simulink library "merge_control_lib"  (Simulink 8.2)
settings: Solver=ode1  StartTime=0.0  StopTime=Inf  FixedStep=0.001  RelTol=1e-3
PostLoadFcn:
  | , if any(exist('dsrtsu_mdlpostloadfcn', 'file') == [2, 3, 6]), try dsrtsu_mdlpostloadfcn('Execute', bdroot); catch fprintf('Error in PostLoadFcn (dsrtsu_mdlpostloadfcn) for model "%s":\n %s\n', bdroot, lasterr); end, end,
libraries: merge_control_lib x6, simulink x4
settings Model: DSRTSU_INTERNAL_RTI_VER=450  DSRTSU_INTERNAL_RTI_TYPE=rti1401  DSRTSU_INTERNAL_RTIFPGA=40  Creator=rushk1  LastModifiedBy=rushk1

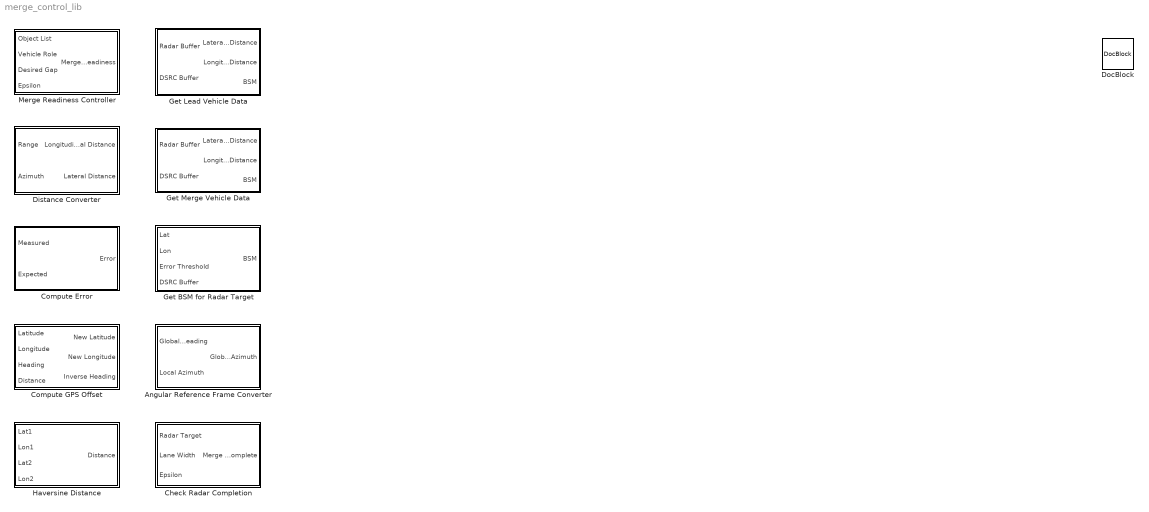
== system merge_control_lib ==
  Angular Reference Frame Converter : Subsystem
  Check Radar Completion : Subsystem
  Compute Error : Subsystem
  Compute GPS Offset : Subsystem
  Distance Converter : Subsystem  TreatAsAtomicUnit=on
      settings: RTWFcnNameOpts=Use subsystem name  RTWFileNameOpts=Use function name
  DocBlock : simulink/Model-Wide Utilities/DocBlock  DocumentType=Text
  Get BSM for Radar Target : Subsystem
  Get Lead Vehicle Data : Subsystem
  Get Merge Vehicle Data : Subsystem
  Haversine Distance : Subsystem
  Merge Readiness Controller : Subsystem

== system merge_control_lib/Angular Reference Frame Converter ==
  Global Heading : Inport
  Local Azimuth : Inport  Port=2
  Degrees in Circle : Constant  Value=360
  Math Function : Math  Operator=mod  OutputSignalType=real  SaturateOnIntegerOverflow=on
  Sum : Sum  Inputs=|++
  Global Azimuth : Outport
  wires:
  Local Azimuth/1 -> Sum/2
  Global Heading/1 -> Sum/1
  Sum/1 -> Math Function/1
  Math Function/1 -> Global Azimuth/1
  Degrees in Circle/1 -> Math Function/2

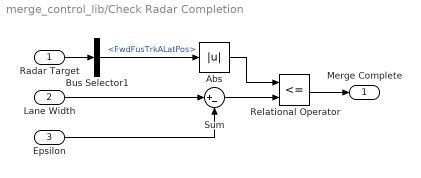
== system merge_control_lib/Check Radar Completion ==
  Radar Target : Inport  OutDataTypeStr=Bus: FusObjectTrackA
  Lane Width : Inport  Port=2  OutDataTypeStr=double
  Epsilon : Inport  Port=3  OutDataTypeStr=double
  Abs : Abs
  Bus Selector1 : BusSelector  OutputSignals=FwdFusTrkALatPos
  Relational Operator : RelationalOperator  Operator=<=  OutDataTypeStr=boolean
  Sum : Sum  Inputs=|+-
  Merge Complete : Outport
  wires:
  Radar Target/1 -> Bus Selector1/1
  Bus Selector1/1 -> Abs/1  "<FwdFusTrkALatPos>"
  Lane Width/1 -> Sum/1
  Relational Operator/1 -> Merge Complete/1
  Abs/1 -> Relational Operator/1
  Sum/1 -> Relational Operator/2
  Epsilon/1 -> Sum/2

== system merge_control_lib/Compute Error ==
  Measured : Inport
  Expected : Inport  Port=2
  Abs : Abs
  Subtract : Sum  Inputs=+-
  Error : Outport
  wires:
  Measured/1 -> Subtract/1
  Expected/1 -> Subtract/2
  Subtract/1 -> Abs/1
  Abs/1 -> Error/1

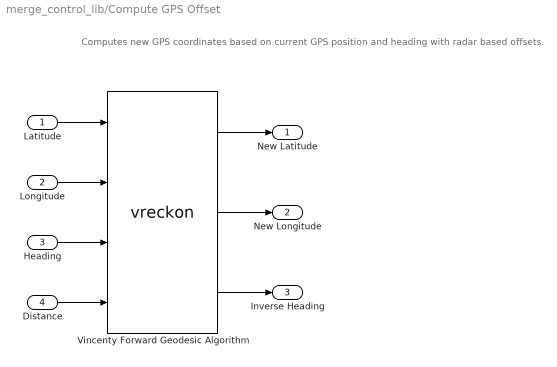
== system merge_control_lib/Compute GPS Offset ==
  note: Computes new GPS coordinates based on current GPS position and heading with radar based offsets.
  Latitude : Inport
  Longitude : Inport  Port=2
  Heading : Inport  Port=3
  Distance : Inport  Port=4
  Vincenty Forward Geodesic Algorithm : M-S-Function  FunctionName=vreckon
  New Latitude : Outport
  New Longitude : Outport  Port=2
  Inverse Heading : Outport  Port=3
  wires:
  Latitude/1 -> Vincenty Forward Geodesic Algorithm/1
  Longitude/1 -> Vincenty Forward Geodesic Algorithm/2
  Distance/1 -> Vincenty Forward Geodesic Algorithm/4
  Heading/1 -> Vincenty Forward Geodesic Algorithm/3
  Vincenty Forward Geodesic Algorithm/1 -> New Latitude/1
  Vincenty Forward Geodesic Algorithm/2 -> New Longitude/1
  Vincenty Forward Geodesic Algorithm/3 -> Inverse Heading/1

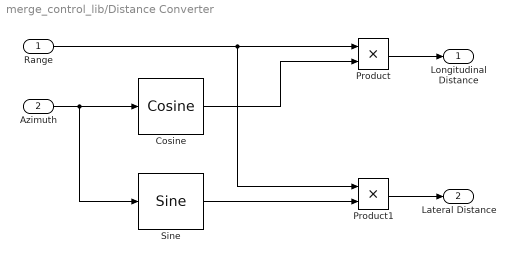
== system merge_control_lib/Distance Converter ==
  Range : Inport
  Azimuth : Inport  Port=2
  Cosine : simulink/Lookup Tables/Cosine  Formula=cos(2*pi*u)  NumDataPoints=(2^5)+1  OutputWordLength=16  InternalRulePriority=Speed
  Product : Product
  Product1 : Product
  Sine : simulink/Lookup Tables/Sine  Formula=sin(2*pi*u)  NumDataPoints=(2^5)+1  OutputWordLength=16  InternalRulePriority=Speed
  Longitudinal Distance : Outport
  Lateral Distance : Outport  Port=2
  wires:
  Product/1 -> Longitudinal Distance/1
  Azimuth/1 -> Sine/1, Cosine/1
  Cosine/1 -> Product/2
  Range/1 -> Product1/1, Product/1
  Product1/1 -> Lateral Distance/1
  Sine/1 -> Product1/2

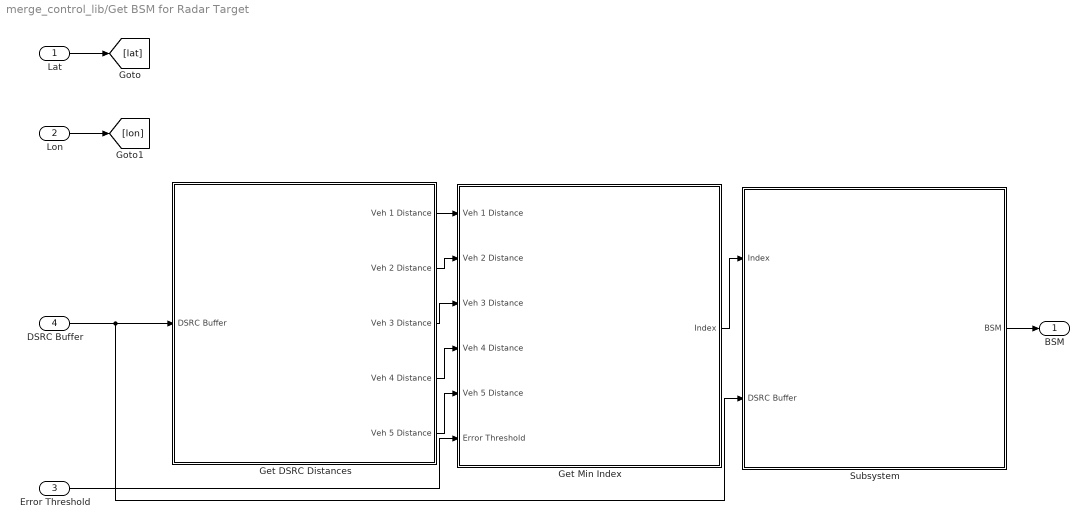
== system merge_control_lib/Get BSM for Radar Target ==
  Lat : Inport
  Lon : Inport  Port=2
  Error Threshold : Inport  Port=3
  DSRC Buffer : Inport  Port=4  OutDataTypeStr=Bus: BSMStoreBus
  Get DSRC Distances : Subsystem
  Get Min Index : Subsystem
  Subsystem : Subsystem
  BSM : Outport
  wires:
  Lat/1 -> [lat]
  Lon/1 -> [lon]
  DSRC Buffer/1 -> Subsystem/2(DSRC Buffer), Get DSRC Distances/1(DSRC Buffer)
  Get DSRC Distances/1(Veh 1 Distance) -> Get Min Index/1(Veh 1 Distance)
  Get DSRC Distances/4(Veh 4 Distance) -> Get Min Index/4(Veh 4 Distance)
  Get DSRC Distances/2(Veh 2 Distance) -> Get Min Index/2(Veh 2 Distance)
  Get DSRC Distances/5(Veh 5 Distance) -> Get Min Index/5(Veh 5 Distance)
  Get DSRC Distances/3(Veh 3 Distance) -> Get Min Index/3(Veh 3 Distance)
  Subsystem/1(BSM) -> BSM/1
  Error Threshold/1 -> Get Min Index/6(Error Threshold)
  Get Min Index/1(Index) -> Subsystem/1(Index)

== system merge_control_lib/Get Lead Vehicle Data ==
  Radar Buffer : Inport
  DSRC Buffer : Inport  Port=2
  Lateral Distance : Outport
  Longitudinal Distance : Outport  Port=2
  BSM : Outport  Port=3

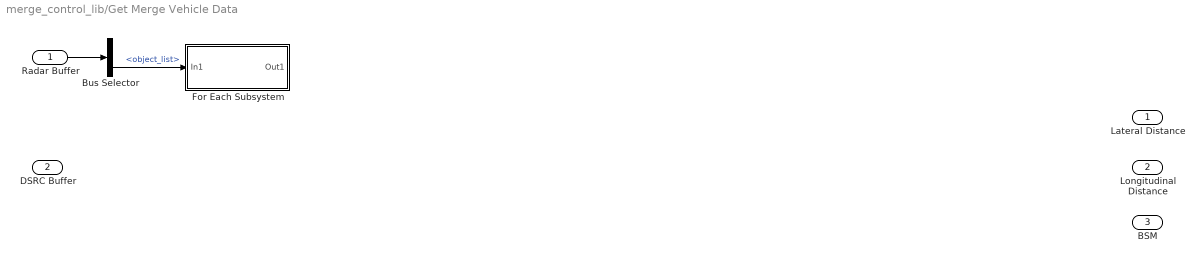
== system merge_control_lib/Get Merge Vehicle Data ==
  Radar Buffer : Inport  OutDataTypeStr=Bus: FusObjectList
  DSRC Buffer : Inport  Port=2
  Bus Selector : BusSelector  OutputSignals=num_objects,object_list
  For Each Subsystem : Subsystem  TreatAsAtomicUnit=on
  Lateral Distance : Outport
  Longitudinal Distance : Outport  Port=2
  BSM : Outport  Port=3
  wires:
  Radar Buffer/1 -> Bus Selector/1
  Bus Selector/2 -> For Each Subsystem/1(In1)  "<object_list>"

== system merge_control_lib/Haversine Distance ==
  note: Computes the Haversine Distance formula between two Lat/Lon pairs
  Lat1 : Inport
  Lon1 : Inport  Port=2
  Lat2 : Inport  Port=3
  Lon2 : Inport  Port=4
  Distance : Outport

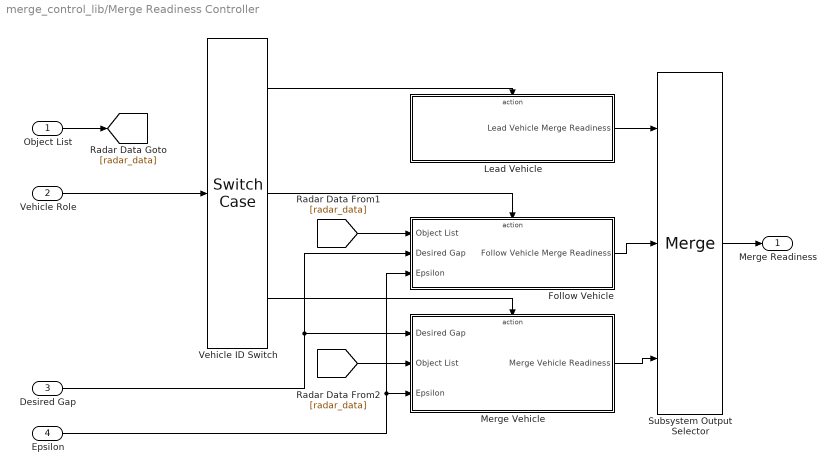
== system merge_control_lib/Merge Readiness Controller ==
  Object List : Inport  OutDataTypeStr=Bus: DetailedObjectList
  Vehicle Role : Inport  Port=2  OutDataTypeStr=Enum: VehicleRoleEnum
  Desired Gap : Inport  Port=3
  Epsilon : Inport  Port=4
  Follow Vehicle : Subsystem  TreatAsAtomicUnit=on
  Lead Vehicle : Subsystem  TreatAsAtomicUnit=on
  Merge Vehicle : Subsystem  TreatAsAtomicUnit=on
  Subsystem Output Selector : Merge  Inputs=3
  Vehicle ID Switch : SwitchCase  CaseConditions={VehicleRoleEnum.LEAD,VehicleRoleEnum.FOLLOW,VehicleRoleEnum.MERGE}  ShowDefaultCase=off
  Merge Readiness : Outport
  wires:
  Lead Vehicle/1(Lead Vehicle Merge Readiness) -> Subsystem Output Selector/1
  Follow Vehicle/1(Follow Vehicle Merge Readiness) -> Subsystem Output Selector/2
  Merge Vehicle/1(Merge Vehicle Readiness) -> Subsystem Output Selector/3
  Vehicle ID Switch/1 -> Lead Vehicle/Action
  Vehicle ID Switch/2 -> Follow Vehicle/Action
  Vehicle ID Switch/3 -> Merge Vehicle/Action
  Vehicle Role/1 -> Vehicle ID Switch/1
  Object List/1 -> [radar_data]
  [radar_data] -> Follow Vehicle/1(Object List)
  Subsystem Output Selector/1 -> Merge Readiness/1
  Desired Gap/1 -> Follow Vehicle/2(Desired Gap), Merge Vehicle/1(Desired Gap)
  [radar_data] -> Merge Vehicle/2(Object List)
  Epsilon/1 -> Merge Vehicle/3(Epsilon), Follow Vehicle/3(Epsilon)

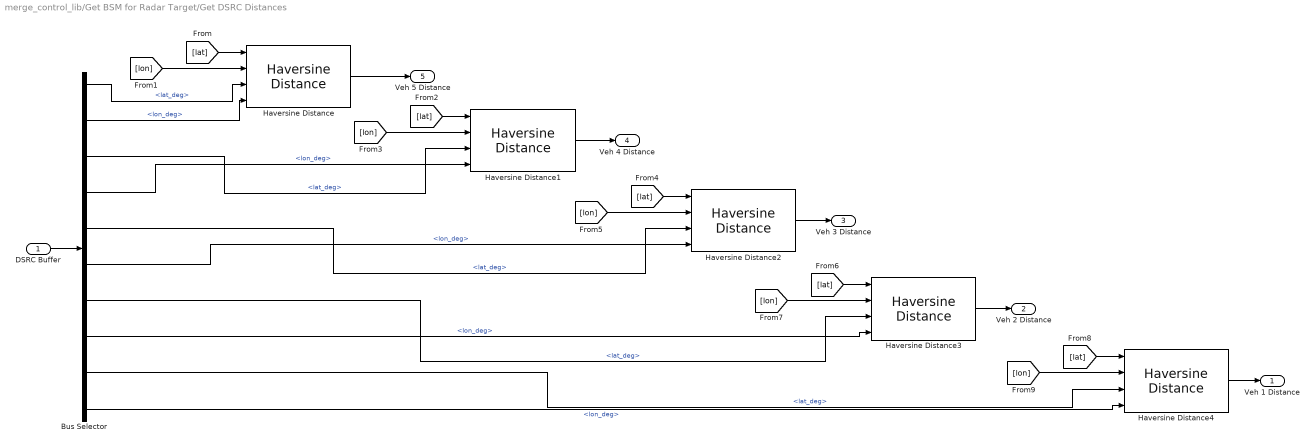
== system merge_control_lib/Get BSM for Radar Target/Get DSRC Distances ==
  DSRC Buffer : Inport
  Bus Selector : BusSelector  OutputSignals=Veh5BSM.lat_deg,Veh5BSM.lon_deg,Veh4BSM.lat_deg,Veh4BSM.lon_deg,Veh3BSM.lat_deg,Veh3BSM.lon_deg,Veh2BSM.lat_deg,Veh2BSM.lon_deg,Veh1BSM.lat_deg,Veh1BSM.lon_deg
  Haversine Distance{,1..4} (5 alike) : merge_control_lib/Haversine Distance
  Veh 1 Distance : Outport
  Veh 2 Distance : Outport  Port=2
  Veh 3 Distance : Outport  Port=3
  Veh 4 Distance : Outport  Port=4
  Veh 5 Distance : Outport  Port=5
  wires:
  DSRC Buffer/1 -> Bus Selector/1
  [lon] -> Haversine Distance/2
  [lat] -> Haversine Distance/1
  Bus Selector/1 -> Haversine Distance/3  "<lat_deg>"
  Bus Selector/2 -> Haversine Distance/4  "<lon_deg>"
  [lon] -> Haversine Distance1/2
  [lat] -> Haversine Distance1/1
  Bus Selector/3 -> Haversine Distance1/3  "<lat_deg>"
  Bus Selector/4 -> Haversine Distance1/4  "<lon_deg>"
  [lon] -> Haversine Distance2/2
  [lat] -> Haversine Distance2/1
  Bus Selector/5 -> Haversine Distance2/3  "<lat_deg>"
  Bus Selector/6 -> Haversine Distance2/4  "<lon_deg>"
  [lon] -> Haversine Distance3/2
  [lat] -> Haversine Distance3/1
  Bus Selector/7 -> Haversine Distance3/3  "<lat_deg>"
  Bus Selector/8 -> Haversine Distance3/4  "<lon_deg>"
  [lon] -> Haversine Distance4/2
  [lat] -> Haversine Distance4/1
  Bus Selector/9 -> Haversine Distance4/3  "<lat_deg>"
  Bus Selector/10 -> Haversine Distance4/4  "<lon_deg>"
  Haversine Distance/1 -> Veh 5 Distance/1
  Haversine Distance1/1 -> Veh 4 Distance/1
  Haversine Distance2/1 -> Veh 3 Distance/1
  Haversine Distance3/1 -> Veh 2 Distance/1
  Haversine Distance4/1 -> Veh 1 Distance/1

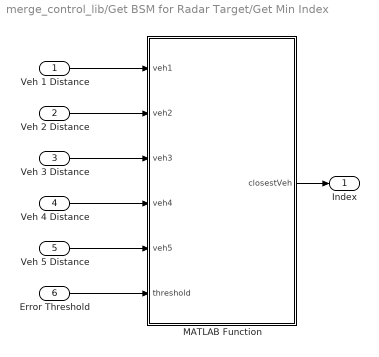
== system merge_control_lib/Get BSM for Radar Target/Get Min Index ==
  Veh 1 Distance : Inport
  Veh 2 Distance : Inport  Port=2
  Veh 3 Distance : Inport  Port=3
  Veh 4 Distance : Inport  Port=4
  Veh 5 Distance : Inport  Port=5
  Error Threshold : Inport  Port=6
  MATLAB Function : MATLAB Function  TreatAsAtomicUnit=on
  Index : Outport
  wires:
  Veh 1 Distance/1 -> MATLAB Function/1(veh1)
  Veh 2 Distance/1 -> MATLAB Function/2(veh2)
  Veh 3 Distance/1 -> MATLAB Function/3(veh3)
  Veh 4 Distance/1 -> MATLAB Function/4(veh4)
  Veh 5 Distance/1 -> MATLAB Function/5(veh5)
  MATLAB Function/1(closestVeh) -> Index/1
  Error Threshold/1 -> MATLAB Function/6(threshold)

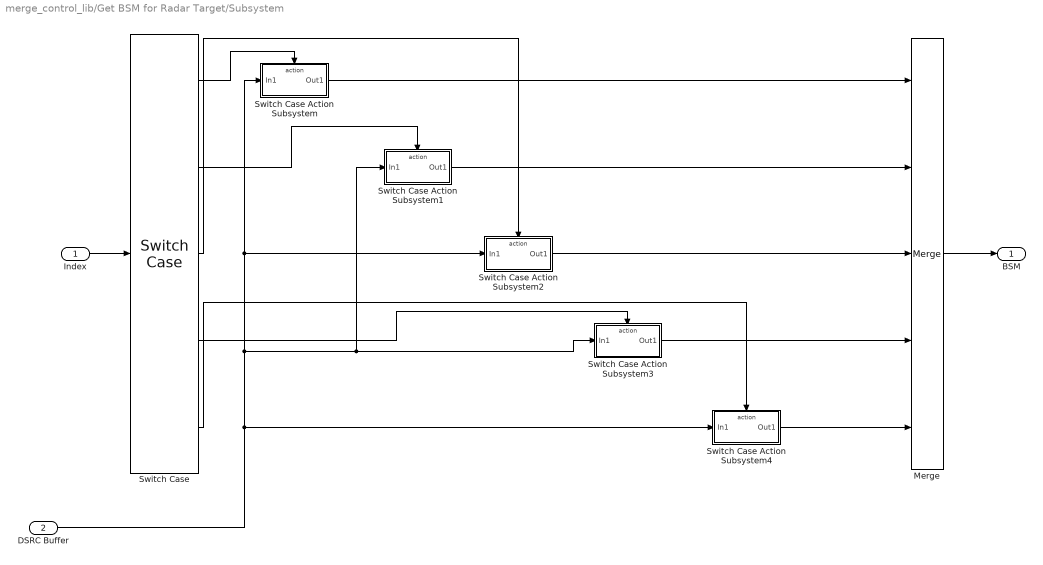
== system merge_control_lib/Get BSM for Radar Target/Subsystem ==
  Index : Inport
  DSRC Buffer : Inport  Port=2
  Merge : Merge  Inputs=5
  Switch Case : SwitchCase  CaseConditions={1,2,3,4,5}  ShowDefaultCase=off
  Switch Case Action Subsystem : Subsystem  TreatAsAtomicUnit=on
  Switch Case Action Subsystem1 : Subsystem  AncestorBlock=merge_control_lib/Get BSM for Radar Target/Subsystem/Switch Case Action Subsystem  TreatAsAtomicUnit=on
  Switch Case Action Subsystem2 : Subsystem  TreatAsAtomicUnit=on
  Switch Case Action Subsystem3 : Subsystem  TreatAsAtomicUnit=on
  Switch Case Action Subsystem4 : Subsystem  TreatAsAtomicUnit=on
  BSM : Outport
  wires:
  Index/1 -> Switch Case/1
  Switch Case/1 -> Switch Case Action Subsystem/Action
  Switch Case/2 -> Switch Case Action Subsystem1/Action
  Switch Case/3 -> Switch Case Action Subsystem2/Action
  Switch Case/4 -> Switch Case Action Subsystem3/Action
  Switch Case/5 -> Switch Case Action Subsystem4/Action
  DSRC Buffer/1 -> Switch Case Action Subsystem4/1(In1), Switch Case Action Subsystem3/1(In1), Switch Case Action Subsystem1/1(In1), Switch Case Action Subsystem2/1(In1), Switch Case Action Subsystem/1(In1)
  Switch Case Action Subsystem/1(Out1) -> Merge/1
  Switch Case Action Subsystem1/1(Out1) -> Merge/2
  Switch Case Action Subsystem2/1(Out1) -> Merge/3
  Switch Case Action Subsystem3/1(Out1) -> Merge/4
  Switch Case Action Subsystem4/1(Out1) -> Merge/5
  Merge/1 -> BSM/1

== system merge_control_lib/Get Merge Vehicle Data/For Each Subsystem ==
  In1 : Inport  Partition=on  PartitionDimension=1  PartitionWidth=1
  Bus Selector : BusSelector  OutputSignals=long_dist_m,long_vel_m_s
  For Each : ForEach  DisableCoverage=on  IndexMode=One-based
  GPS/Radar Target Unity : merge_control_lib/GPS//Radar Target Unity
  Out1 : Outport  ConcatenationDimension=1
  wires:
  In1/1 -> Bus Selector/1

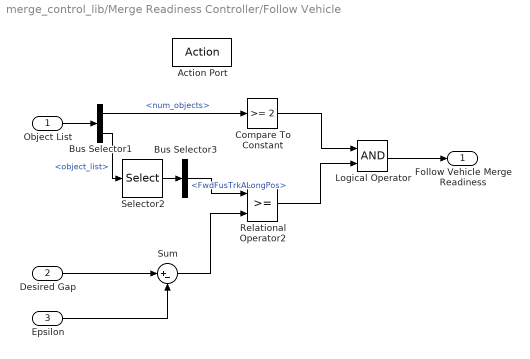
== system merge_control_lib/Merge Readiness Controller/Follow Vehicle ==
  Object List : Inport  OutDataTypeStr=Bus: DetailedObjectList
  Desired Gap : Inport  Port=2
  Epsilon : Inport  Port=3
  Action Port : ActionPort  ActionType=case
  Bus Selector1 : BusSelector  OutputSignals=num_objects,object_list
  Bus Selector3 : BusSelector  OutputSignals=FwdFusTrkALongPos
  Compare To Constant : simulink/Logic and Bit Operations/Compare To Constant  relop=>=  const=2  OutDataTypeStr=boolean
  Logical Operator : Logic  AllPortsSameDT=off  OutDataTypeStr=boolean
  Relational Operator2 : RelationalOperator  OutDataTypeStr=boolean
  Selector2 : Selector  InputPortWidth=4  IndexOptions=Index vector (dialog)  Indices=1  OutputSizes=1
  Sum : Sum  Inputs=|+-
  Follow Vehicle Merge Readiness : Outport
  wires:
  Object List/1 -> Bus Selector1/1
  Relational Operator2/1 -> Logical Operator/2
  Desired Gap/1 -> Sum/1
  Bus Selector1/2 -> Selector2/1  "<object_list>"
  Bus Selector3/1 -> Relational Operator2/1  "<FwdFusTrkALongPos>"
  Selector2/1 -> Bus Selector3/1
  Sum/1 -> Relational Operator2/2
  Epsilon/1 -> Sum/2
  Bus Selector1/1 -> Compare To Constant/1  "<num_objects>"
  Compare To Constant/1 -> Logical Operator/1
  Logical Operator/1 -> Follow Vehicle Merge Readiness/1

== system merge_control_lib/Merge Readiness Controller/Lead Vehicle ==
  Action Port : ActionPort  ActionType=case
  Always Ready : Constant  Value=true
  Lead Vehicle Merge Readiness : Outport
  wires:
  Always Ready/1 -> Lead Vehicle Merge Readiness/1

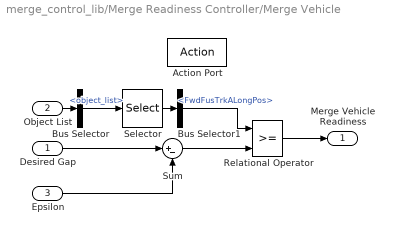
== system merge_control_lib/Merge Readiness Controller/Merge Vehicle ==
  Desired Gap : Inport
  Object List : Inport  Port=2  OutDataTypeStr=Bus: DetailedObjectList
  Epsilon : Inport  Port=3
  Action Port : ActionPort  ActionType=case
  Bus Selector : BusSelector  OutputSignals=object_list
  Bus Selector1 : BusSelector  OutputSignals=FwdFusTrkALongPos
  Relational Operator : RelationalOperator  OutDataTypeStr=boolean
  Selector : Selector  InputPortWidth=4  IndexOptions=Index vector (dialog)  Indices=1  OutputSizes=1
  Sum : Sum  Inputs=|+-
  Merge Vehicle Readiness : Outport
  wires:
  Object List/1 -> Bus Selector/1
  Bus Selector/1 -> Selector/1  "<object_list>"
  Desired Gap/1 -> Sum/1
  Selector/1 -> Bus Selector1/1
  Relational Operator/1 -> Merge Vehicle Readiness/1
  Bus Selector1/1 -> Relational Operator/1  "<FwdFusTrkALongPos>"
  Sum/1 -> Relational Operator/2
  Epsilon/1 -> Sum/2

== system merge_control_lib/Get BSM for Radar Target/Subsystem/Switch Case Action Subsystem ==
  In1 : Inport
  Action Port : ActionPort  ActionType=case
  Bus Selector : BusSelector  OutputSignals=Veh1BSM
  Out1 : Outport
  wires:
  In1/1 -> Bus Selector/1
  Bus Selector/1 -> Out1/1  "<Veh1BSM>"

== system merge_control_lib/Get BSM for Radar Target/Subsystem/Switch Case Action Subsystem1 ==
  In1 : Inport
  Action Port : ActionPort
  Bus Selector : BusSelector  OutputSignals=Veh2BSM
  Out1 : Outport
  wires:
  Bus Selector/1 -> Out1/1  "<Veh2BSM>"
  In1/1 -> Bus Selector/1

== system merge_control_lib/Get BSM for Radar Target/Subsystem/Switch Case Action Subsystem2 ==
  In1 : Inport
  Action Port : ActionPort  ActionType=case
  Bus Selector : BusSelector  OutputSignals=Veh3BSM
  Out1 : Outport
  wires:
  In1/1 -> Bus Selector/1
  Bus Selector/1 -> Out1/1  "<Veh3BSM>"

== system merge_control_lib/Get BSM for Radar Target/Subsystem/Switch Case Action Subsystem3 ==
  In1 : Inport
  Action Port : ActionPort  ActionType=case
  Bus Selector : BusSelector  OutputSignals=Veh4BSM
  Out1 : Outport
  wires:
  In1/1 -> Bus Selector/1
  Bus Selector/1 -> Out1/1  "<Veh4BSM>"

== system merge_control_lib/Get BSM for Radar Target/Subsystem/Switch Case Action Subsystem4 ==
  In1 : Inport
  Action Port : ActionPort  ActionType=case
  Bus Selector : BusSelector  OutputSignals=Veh5BSM
  Out1 : Outport
  wires:
  In1/1 -> Bus Selector/1
  Bus Selector/1 -> Out1/1  "<Veh5BSM>"

== matlab function Get BSM for Radar Target/Get Min Index/MATLAB Function ==
  data: veh1 input double; closestVeh output double; veh2 input double; veh3 input double; veh4 input double; veh5 input double; threshold input double
% Takes in 5 distances and returns the index (vehicle ID) of the smallest
% one
function closestVeh = fcn(veh1, veh2, veh3, veh4, veh5, threshold)
%#codegen

a = [veh1, veh2, veh3, veh4, veh5];
minDist = Inf;
minIdx = -1;
len = size(a);
for n = 1:len(1)
    if (a(n) <= minDist) && (a(n) <= threshold)
        minDist = a(n);
        minIdx = n;
    end
end

closestVeh = minIdx;
